simulink model "StateMachineWithBatchEvents"  (R2021b)
settings: Solver=VariableStepAuto  StartTime=0.0  StopTime=10.0  RelTol=1e-3
model workspace (MATLAB code in the model file):
  | % Add the class folders into the path.
  | addpath model
  | addpath utils
  | 
  | %% Loading data from files.
  | % Data for supervisor 1.
  | utils = StateMachineUtils;
  | 
  | % From TCT: Load all events' number.
  | utils = utils.loadEventsInAds('resources/tct/ALLEVENT.ADS');
  | 
  | % From TCT: Disabled events in each state.
  | utils = utils.loadDisabledEventsInPdt('resources/tct/supervisor1/DATA_SIMSUP1_MG1.PDT');
  | 
  | % From TCT: Transition matrix.
  | utils = utils.loadTransitionsInAds('resources/tct/supervisor1/SIMSUP1_MG1.ADS');
  | 
  | % Parameters for the block.
  | encodedStates = StateEncoder.encode(utils.statesArray);
  | 
  | transitions = utils.transitions;
  | 
  | allEvents = utils.eventsArray;
settings Model: Creator=andrerangel  LastModifiedBy=andrerangel

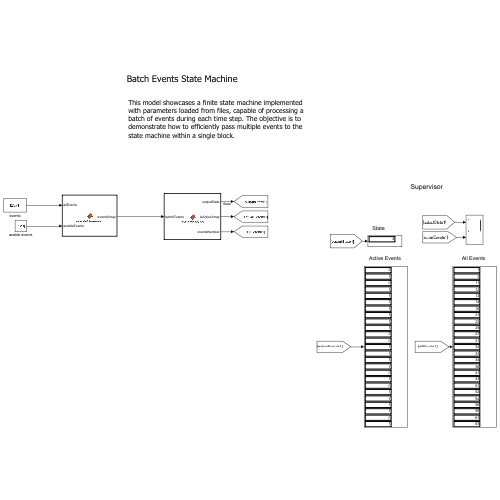
[thumbnail: Simulink's stored preview of the top-level diagram]
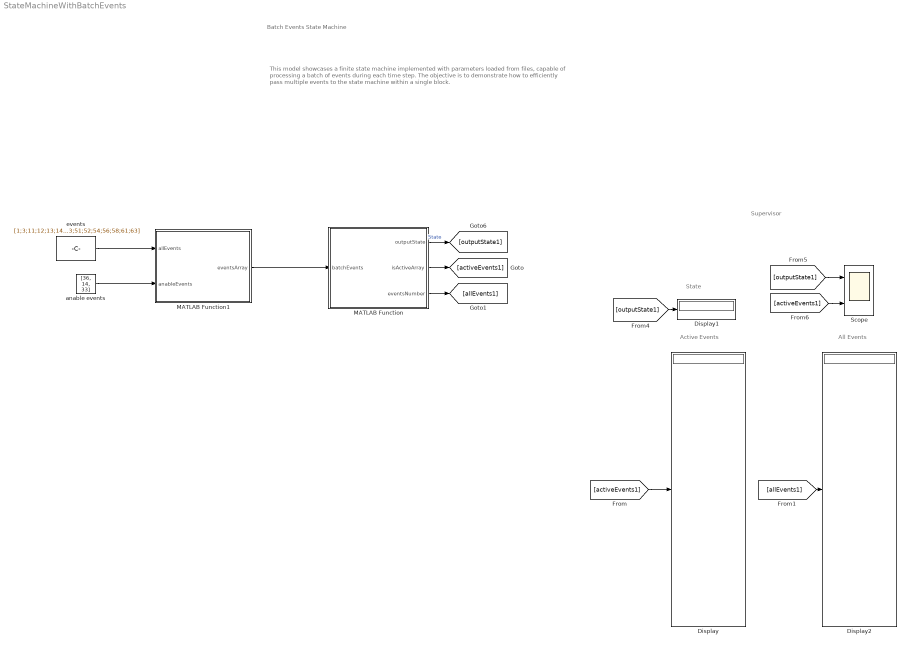
== system StateMachineWithBatchEvents ==
  note: Active Events
  note: Supervisor
  note: This model showcases a finite state machine implemented with parameters loaded from files, capable of processing a batch of events during each time step. The objective is to demonstrate how to efficiently pass multiple events to the state machine within a single block.
  note: State
  note: All Events
  note: Batch Events State Machine
  Display : Display
  Display1 : Display
  Display2 : Display
  MATLAB Function : MATLAB Function  TreatAsAtomicUnit=on
  MATLAB Function1 : MATLAB Function  TreatAsAtomicUnit=on
  Scope : Scope  NumInputPorts=2
  anable events : Constant  Value=[36, 14, 33]
  events : Constant  Value=[1;3;11;12;13;14;16;21;23;25;27;31;32;33;34;36;41;43;51;52;54;56;58;61;63]
  wires:
  MATLAB Function/1(outputState) -> [outputState1]  "State"
  MATLAB Function/3(eventsNumber) -> [allEvents1]
  [outputState1] -> Scope/1
  [activeEvents1] -> Scope/2
  MATLAB Function/2(isActiveArray) -> [activeEvents1]
  [allEvents1] -> Display2/1
  [activeEvents1] -> Display/1
  [outputState1] -> Display1/1
  events/1 -> MATLAB Function1/1(allEvents)
  anable events/1 -> MATLAB Function1/2(anableEvents)
  MATLAB Function1/1(eventsArray) -> MATLAB Function/1(batchEvents)

== matlab function StateMachineWithBatchEvents/MATLAB Function1 ==
  data: allEvents input; anableEvents input; eventsArray output
function eventsArray = eventsGenerator(allEvents, anableEvents)

[~, indexes] = ismember(anableEvents, allEvents);

eventsArray = zeros(length(allEvents), 1);

eventsArray(indexes) = 1;

== matlab function StateMachineWithBatchEvents/MATLAB Function ==
  data: batchEvents input; outputState output size=[1 1]; isActiveArray output; eventsNumber output; allEvents parameter; transitions parameter; encodedStates parameter
function [outputState, isActiveArray, eventsNumber] = stateMachine( ...
    batchEvents, ...
    allEvents, ...
    transitions, ...
    encodedStates)
% State Machine with parameters from files.
% Receives a batch of events and process one event at time, starting with
% the event of index 1.
% batchEvents: array with 0s and 1s where 1 is the enabled event while 0,
% is disabled event;
% allEvents: numbers of the events;
% transitions: matrix of transitions;
% encodedStates: Encoded states array to be decoded before the pass it to
% StateMachines as an argument.

% Initialize a persistent object. Its value will not be erased as this
% block finishes.
persistent stateMachine

% Assign the persistent object to the StateMachine class with data passed
% as parameters.
if (isempty(stateMachine))
    statesArray = StateEncoder.decode(encodedStates);                        
    stateMachine = StateMachine(statesArray, transitions, allEvents);
end

anabledEvents = allEvents(logical(batchEvents));

% loop through an array of events:
for i=1:length(anabledEvents)
    stateMachine.inputEvent = anabledEvents(i);
end
outputState = stateMachine.currentState.number;
isActiveArray = stateMachine.currentState.activeEvents;
eventsNumber = stateMachine.eventsArray;
